simulink model "State_feedback_system"  (R2018b)
settings: Solver=ode15s  StartTime=0.0  StopTime=0.1  FixedStep=0.01  RelTol=1e-3
values from neighbouring files (symbols this model uses):
  A = double(A)    [Linearization.m]    (also in findK_emtiazi.m = [1 2 0; 0 -1 3; 0 1 -1])
  B = double(B)    [Linearization.m]
  C = [1 0 0 0 ; 0 1 0 0 ]    [Linearization.m]    (also in findK_emtiazi.m = [0 1 0])
  k = place(A,B,pc)    [Linearization.m]
settings Model: Creator=Mr.Hallajiyan  LastModifiedBy=sepehr
settings OptimizationCC: LifeSpan=inf
settings DebuggingCC: LibraryContextMissingDiagnostic=none  SFExecutionAtInitializationDiag=none
settings SFSimCC: SimUseLocalCustomCode=off
settings RTWCC: RTWUseLocalCustomCode=off
settings CodeAppCC: StateflowObjectComments=on

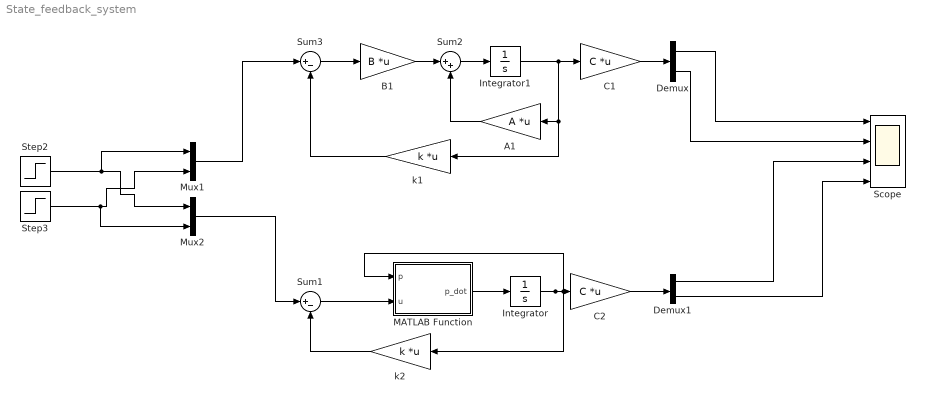
== system State_feedback_system ==
  A1 : Gain  Gain=A  Multiplication=Matrix(K*u) (u vector)
  B1 : Gain  Gain=B  Multiplication=Matrix(K*u) (u vector)
  C1 : Gain  Gain=C  Multiplication=Matrix(K*u) (u vector)
  C2 : Gain  Gain=C  Multiplication=Matrix(K*u) (u vector)
  Demux : Demux  Outputs=2
  Demux1 : Demux  Outputs=2
  Integrator : Integrator
  Integrator1 : Integrator
  MATLAB Function : MATLAB Function  TreatAsAtomicUnit=on
  Mux1 : Mux  Inputs=2
  Mux2 : Mux  Inputs=2
  Scope : Scope  NumInputPorts=4
  Step2 : Step  Time=0  SampleTime=0.0001
  Step3 : Step  Time=0  After=1.2  SampleTime=0.001
  Sum1 : Sum  Inputs=|+-
  Sum2 : Sum  Inputs=|++
  Sum3 : Sum  Inputs=|+-
  k1 : Gain  Gain=k  Multiplication=Matrix(K*u) (u vector)
  k2 : Gain  Gain=k  Multiplication=Matrix(K*u) (u vector)
  wires:
  Demux/2 -> Scope/2
  Demux/1 -> Scope/1
  Sum1/1 -> MATLAB Function/2(u)
  C2/1 -> Demux1/1
  Integrator/1 -> k2/1, MATLAB Function/1(p), C2/1
  MATLAB Function/1(p_dot) -> Integrator/1
  Sum2/1 -> Integrator1/1
  Integrator1/1 -> k1/1, A1/1, C1/1
  C1/1 -> Demux/1
  B1/1 -> Sum2/1
  A1/1 -> Sum2/2
  k2/1 -> Sum1/2
  Mux2/1 -> Sum1/1
  Step2/1 -> Mux1/1, Mux2/1
  Step3/1 -> Mux2/2, Mux1/2
  Demux1/1 -> Scope/3
  Demux1/2 -> Scope/4
  k1/1 -> Sum3/2
  Mux1/1 -> Sum3/1
  Sum3/1 -> B1/1

== matlab function State_feedback_system/MATLAB Function ==
  settings: updateMethod=DISCRETE
  data: p input; u input; p_dot output
function p_dot = fcn(p,u)

a1 = 6.11e-3;
a2 = -2.89e-3;
a3 = -4.24e-3;
a4 = 3.01e-3;
a5 = 2.05e-3;
a6 = 1.92e-3;
a7 = 1.60e-3;
a8 = -8.32e-3;
bw = 30;
cw = 1500;
d1 = 0;
d2 = 0;

p1 = p(1);
p2 = p(2);
p3 = p(3);
p4 = p(4);

M = [a1 + a2*cos(2*p2) + a3*sin(2*p2) + a4*cos(p2) + a5*sin(p2) 0; 0 a6];
M_inv = inv(M);
V = [-2*a1*p3*p4*sin(2*p2) + 2*a3*p3*p4*cos(2*p2) + a4*p3*p4*cos(p2) - a5*p3*p4*sin(p2) ; 
    2*a2*(p3)^2*cos(p2)*sin(p2) - a3*(p3)^2*cos(p2) - 0.5*a4*(p3)^2*cos(p2) + 0.5*a5*(p3)^2*sin(p2) + a7*sin(p2) + a8*cos(p2)];
f = bw*[p3;p4] + cw*[p1;p2];
%u = [u1 ; u2];
d = [d1 ; d2];
C = [1 0 0 0 ; 0 1 0 0 ];


x1_dot = [p3 ; p4];
x2_dot = -M_inv*V - M_inv*f + M_inv*u + M_inv*d;

p_dot = [x1_dot ; x2_dot];
